simulink model "Ejercicio_Inestable_simu"  (R2021a)
settings: Solver=VariableStepAuto  StartTime=0.0  StopTime=10.0  RelTol=1e-3
values from neighbouring files (symbols this model uses):
  A = [-2 -1; 0 -4]    [Control_Integral.m]    (also in Controlabilidad.m = P.a; Ejemplo_filminas.m = SS.A; Ejercicio_Inestable.m = [100, 0; 160, 200]; Ejercicio_Valvulas.m = double(A))
  B = [1; 0]    [Control_Integral.m]    (also in Controlabilidad.m = P.b; Ejemplo_filminas.m = SS.B; Ejercicio_Inestable.m = [70; 160]; Ejercicio_Valvulas.m = double(B))
  C = [1 1]    [Control_Integral.m]    (also in Controlabilidad.m = P.c; Ejemplo_filminas.m = SS.C; Ejercicio_Inestable.m = [1, 1]; Ejercicio_Valvulas.m = double(C))
  D = 0    [Control_Integral.m]    (also in Controlabilidad.m = P.d; Ejemplo_filminas.m = SS.D; Ejercicio_Inestable.m = 1; Ejercicio_Valvulas.m = double(D))
  K = [p1-a1 p2-a2] * Wrm * inv(Wr)    [Controlabilidad.m]    (also in Ejemplo_filminas.m; Ejercicio_Inestable.m = [p1 - a1, p2 - a2] * Wrm * inv(Wr); Ejercicio_Valvulas.m = Ka(1:order(P)); realimentacion_ee.m = acker(A, B, [-10 -10]))
  K_nuevo = Ka(1:order(P))    [Ejemplo_filminas.m]    (also in Ejercicio_Inestable.m = Ka(1:2))
  kf = -1/(C*inv(A - B*K) * B)    [Controlabilidad.m]    (also in Ejemplo_filminas.m = -1/(Ccl * inv(Acl)*Bcl); Ejercicio_Inestable.m = 1/(-(C - D*K) * inv(A - B*K) * B + D); realimentacion_ee.m = 10)
  ki = 10    [Control_Integral.m]    (also in Ejemplo_filminas.m = - Ka(end); Ejercicio_Inestable.m = - Ka(end); Ejercicio_Valvulas.m = - Ka(end))
  L = zpk(ceros, polos, ganancia)    [Ejemplo_filminas.m]    (also in Ejercicio_Inestable.m = inv(Wo) * Wom * [l1 - a1; l2 - a2]; Observabilidad.m = [18; 99]; realimentacion_ee.m = [18; 99])
libraries: cstblocks x1
settings Model: Creator=Santiago  LastModifiedBy=Santiago

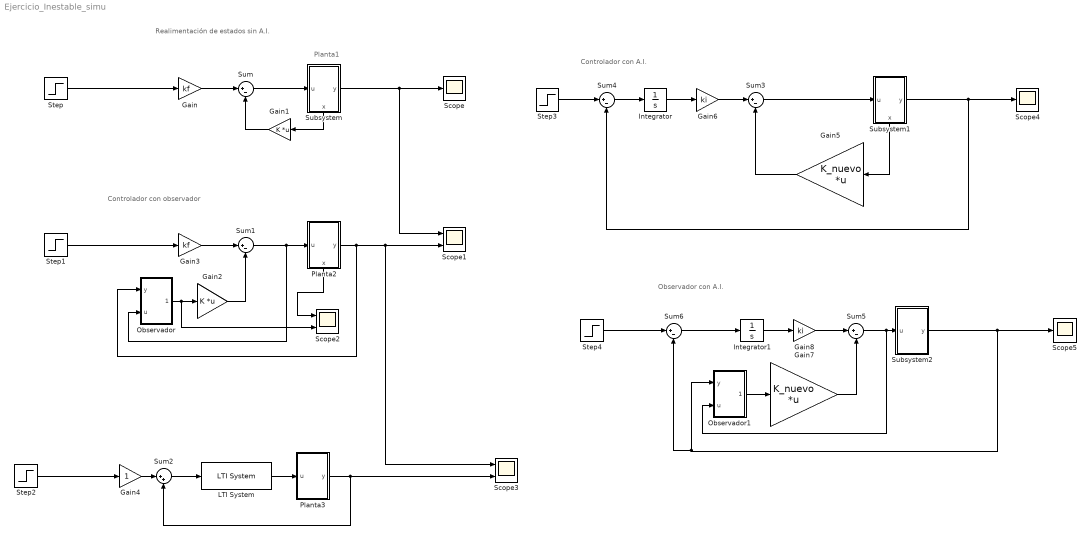
== system Ejercicio_Inestable_simu ==
  note: Observador con A.I.
  note: Controlador con A.I.
  note: Controlador con observador
  note: Realimentación de estados sin A.I.
  note: Planta1
  Gain : Gain  Gain=kf
  Gain1 : Gain  Gain=K  Multiplication=Matrix(K*u) (u vector)
  Gain2 : Gain  Gain=K  Multiplication=Matrix(K*u) (u vector)
  Gain3 : Gain  Gain=kf
  Gain4 : Gain
  Gain5 : Gain  Gain=K_nuevo  Multiplication=Matrix(K*u) (u vector)
  Gain6 : Gain  Gain=ki
  Gain7 : Gain  Gain=K_nuevo  Multiplication=Matrix(K*u) (u vector)
  Gain8 : Gain  Gain=ki
  Integrator : Integrator
  Integrator1 : Integrator
  LTI System : cstblocks/LTI System  sys=rsys  IC=[]
  Observador : Subsystem
  Observador1 : Subsystem
  Planta2 : Subsystem
      settings: PortSchema="{\"entries\":[{\"content\":{\"sides\":[{\"content\":{\"connectorIds\":[\"In1\"]},\"type\":\"ConnectorPlacement.EquallySpacedRectSide\",\"uuid\":\"42671557-4276-46e4-ad8c-bf843df94049\"},{\"content\":{\"connectorIds\":[\"Out1\"],\"side\":\"RIGHT\"},\"type\":\"ConnectorPlacement.EquallySpacedRectSide\",\"uuid\":\"cb79af1c-2dea-4382-b5e6-be31f4841be6\"},{\"content\":{\"connectorIds\":[],\"side\":\"TOP\"},\"type\":\"ConnectorPlacement.EquallySpacedRectSide\",\"uuid\":\"60d3f2a7-7810-4feb-a004-3efb06eed614\"},{\"content\":{\"connectorIds\":[\"Out2\"],\"side\":\"BOTTOM\"},\"type\":\"ConnectorPlacement.EquallySpacedRectSide\",\"uuid\":\"95700307-25c5-43ae-b0f1-57f7147fd329\"}]},\"type\":\"ConnectorPlacement.EquallySpacedConnector\",\"uuid\":\"693bd3af-f156-43df-9cc2-6d7d4d502922\"}],\"packageUris\":[\"http://schema.mathworks.com/mf0/Connector/R2020b\"],\"version\":\"1.0\"}"
  Planta3 : Subsystem
  Scope : Scope
  Scope1 : Scope  NumInputPorts=2
  Scope2 : Scope  NumInputPorts=2
  Scope3 : Scope  NumInputPorts=2
  Scope4 : Scope
  Scope5 : Scope
  Step{,1..4} (5 alike) : Step  SampleTime=0
  Subsystem : Subsystem
      settings: PortSchema="{\"entries\":[{\"content\":{\"sides\":[{\"content\":{\"connectorIds\":[\"In1\"]},\"type\":\"ConnectorPlacement.EquallySpacedRectSide\",\"uuid\":\"42671557-4276-46e4-ad8c-bf843df94049\"},{\"content\":{\"connectorIds\":[\"Out1\"],\"side\":\"RIGHT\"},\"type\":\"ConnectorPlacement.EquallySpacedRectSide\",\"uuid\":\"cb79af1c-2dea-4382-b5e6-be31f4841be6\"},{\"content\":{\"connectorIds\":[],\"side\":\"TOP\"},\"type\":\"ConnectorPlacement.EquallySpacedRectSide\",\"uuid\":\"60d3f2a7-7810-4feb-a004-3efb06eed614\"},{\"content\":{\"connectorIds\":[\"Out2\"],\"side\":\"BOTTOM\"},\"type\":\"ConnectorPlacement.EquallySpacedRectSide\",\"uuid\":\"9a7d0ef6-39ec-42a5-a60a-a43f88d1fbb1\"}]},\"type\":\"ConnectorPlacement.EquallySpacedConnector\",\"uuid\":\"693bd3af-f156-43df-9cc2-6d7d4d502922\"}],\"packageUris\":[\"http://schema.mathworks.com/mf0/Connector/R2020b\"],\"version\":\"1.0\"}"
  Subsystem1 : Subsystem
      settings: PortSchema="{\"entries\":[{\"content\":{\"sides\":[{\"content\":{\"connectorIds\":[\"In1\"]},\"type\":\"ConnectorPlacement.EquallySpacedRectSide\",\"uuid\":\"42671557-4276-46e4-ad8c-bf843df94049\"},{\"content\":{\"connectorIds\":[\"Out1\"],\"side\":\"RIGHT\"},\"type\":\"ConnectorPlacement.EquallySpacedRectSide\",\"uuid\":\"cb79af1c-2dea-4382-b5e6-be31f4841be6\"},{\"content\":{\"connectorIds\":[],\"side\":\"TOP\"},\"type\":\"ConnectorPlacement.EquallySpacedRectSide\",\"uuid\":\"60d3f2a7-7810-4feb-a004-3efb06eed614\"},{\"content\":{\"connectorIds\":[\"Out2\"],\"side\":\"BOTTOM\"},\"type\":\"ConnectorPlacement.EquallySpacedRectSide\",\"uuid\":\"9a7d0ef6-39ec-42a5-a60a-a43f88d1fbb1\"}]},\"type\":\"ConnectorPlacement.EquallySpacedConnector\",\"uuid\":\"693bd3af-f156-43df-9cc2-6d7d4d502922\"}],\"packageUris\":[\"http://schema.mathworks.com/mf0/Connector/R2020b\"],\"version\":\"1.0\"}"
  Subsystem2 : Subsystem
  Sum{,1,3..6} (6 alike) : Sum  Inputs=|+-
  Sum2 : Sum  Inputs=|++
  wires:
  Subsystem/1(y) -> Scope1/1, Scope/1
  Subsystem/2(x) -> Gain1/1
  Sum/1 -> Subsystem/1(u)
  Gain/1 -> Sum/1
  Step/1 -> Gain/1
  Gain1/1 -> Sum/2
  Observador/1(x_estim) -> Scope2/2, Gain2/1
  Gain2/1 -> Sum1/2
  Sum1/1 -> Observador/2(u), Planta2/1(u)
  Planta2/1(y) -> Observador/1(y), Scope3/1, Scope1/2
  Step1/1 -> Gain3/1
  Gain3/1 -> Sum1/1
  Planta2/2(x) -> Scope2/1
  Step2/1 -> Gain4/1
  Planta3/1(y) -> Sum2/2, Scope3/2
  Sum2/1 -> LTI System/1
  Gain4/1 -> Sum2/1
  LTI System/1 -> Planta3/1(u)
  Gain5/1 -> Sum3/2
  Gain6/1 -> Sum3/1
  Integrator/1 -> Gain6/1
  Sum4/1 -> Integrator/1
  Step3/1 -> Sum4/1
  Subsystem1/2(x) -> Gain5/1
  Sum3/1 -> Subsystem1/1(u)
  Subsystem1/1(y) -> Sum4/2, Scope4/1
  Gain8/1 -> Sum5/1
  Integrator1/1 -> Gain8/1
  Observador1/1(x_estim) -> Gain7/1
  Gain7/1 -> Sum5/2
  Sum5/1 -> Observador1/2(u), Subsystem2/1(u)
  Subsystem2/1(y) -> Sum6/2, Observador1/1(y), Scope5/1
  Step4/1 -> Sum6/1
  Sum6/1 -> Integrator1/1

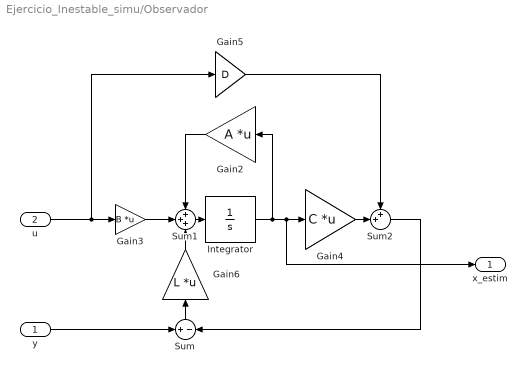
== system Ejercicio_Inestable_simu/Observador ==
  y : Inport
  u : Inport  Port=2
  Gain2 : Gain  Gain=A  Multiplication=Matrix(K*u) (u vector)
  Gain3 : Gain  Gain=B  Multiplication=Matrix(K*u)
  Gain4 : Gain  Gain=C  Multiplication=Matrix(K*u) (u vector)
  Gain5 : Gain  Gain=D
  Gain6 : Gain  Gain=L  Multiplication=Matrix(K*u) (u vector)
  Integrator : Integrator
  Sum : Sum  Inputs=+|-
  Sum1 : Sum  Inputs=+++
  Sum2 : Sum  Inputs=++|
  x_estim : Outport
  wires:
  Sum2/1 -> Sum/2
  Integrator/1 -> Gain4/1, x_estim/1, Gain2/1
  Gain5/1 -> Sum2/1
  Gain3/1 -> Sum1/2
  Gain4/1 -> Sum2/2
  u/1 -> Gain5/1, Gain3/1
  Sum1/1 -> Integrator/1
  Gain2/1 -> Sum1/1
  y/1 -> Sum/1
  Sum/1 -> Gain6/1
  Gain6/1 -> Sum1/3

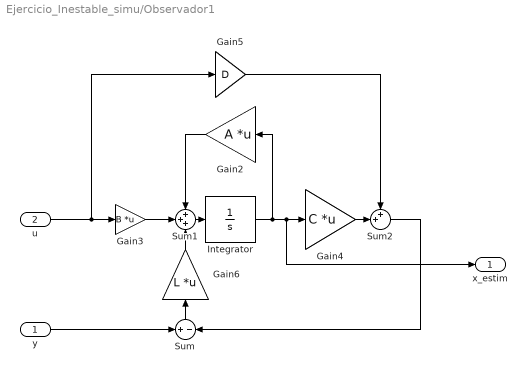
== system Ejercicio_Inestable_simu/Observador1 ==
  y : Inport
  u : Inport  Port=2
  Gain2 : Gain  Gain=A  Multiplication=Matrix(K*u) (u vector)
  Gain3 : Gain  Gain=B  Multiplication=Matrix(K*u)
  Gain4 : Gain  Gain=C  Multiplication=Matrix(K*u) (u vector)
  Gain5 : Gain  Gain=D
  Gain6 : Gain  Gain=L  Multiplication=Matrix(K*u) (u vector)
  Integrator : Integrator
  Sum : Sum  Inputs=+|-
  Sum1 : Sum  Inputs=+++
  Sum2 : Sum  Inputs=++|
  x_estim : Outport
  wires:
  Sum2/1 -> Sum/2
  Integrator/1 -> Gain4/1, x_estim/1, Gain2/1
  Gain5/1 -> Sum2/1
  Gain3/1 -> Sum1/2
  Gain4/1 -> Sum2/2
  u/1 -> Gain5/1, Gain3/1
  Sum1/1 -> Integrator/1
  Gain2/1 -> Sum1/1
  y/1 -> Sum/1
  Sum/1 -> Gain6/1
  Gain6/1 -> Sum1/3

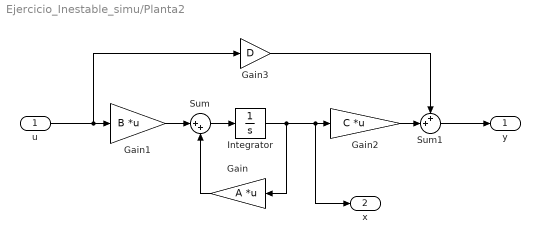
== system Ejercicio_Inestable_simu/Planta2 ==
  u : Inport
  Gain : Gain  Gain=A  Multiplication=Matrix(K*u) (u vector)
  Gain1 : Gain  Gain=B  Multiplication=Matrix(K*u) (u vector)
  Gain2 : Gain  Gain=C  Multiplication=Matrix(K*u) (u vector)
  Gain3 : Gain  Gain=D
  Integrator : Integrator
  Sum : Sum  Inputs=|++
  Sum1 : Sum  Inputs=++|
  y : Outport
  x : Outport  Port=2
  wires:
  Integrator/1 -> x/1, Gain2/1, Gain/1
  Gain/1 -> Sum/2
  Sum/1 -> Integrator/1
  Gain2/1 -> Sum1/2
  u/1 -> Gain3/1, Gain1/1
  Sum1/1 -> y/1
  Gain3/1 -> Sum1/1
  Gain1/1 -> Sum/1

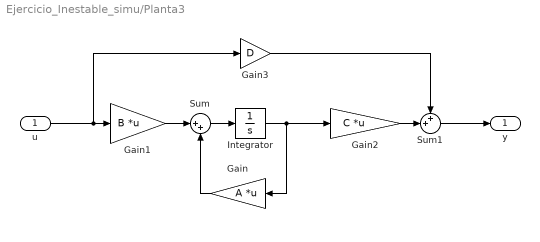
== system Ejercicio_Inestable_simu/Planta3 ==
  u : Inport
  Gain : Gain  Gain=A  Multiplication=Matrix(K*u) (u vector)
  Gain1 : Gain  Gain=B  Multiplication=Matrix(K*u) (u vector)
  Gain2 : Gain  Gain=C  Multiplication=Matrix(K*u) (u vector)
  Gain3 : Gain  Gain=D
  Integrator : Integrator
  Sum : Sum  Inputs=|++
  Sum1 : Sum  Inputs=++|
  y : Outport
  wires:
  Integrator/1 -> Gain2/1, Gain/1
  Gain/1 -> Sum/2
  Sum/1 -> Integrator/1
  Gain2/1 -> Sum1/2
  u/1 -> Gain3/1, Gain1/1
  Sum1/1 -> y/1
  Gain3/1 -> Sum1/1
  Gain1/1 -> Sum/1

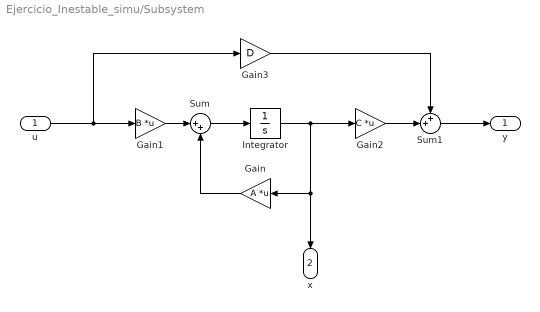
== system Ejercicio_Inestable_simu/Subsystem ==
  u : Inport
  Gain : Gain  Gain=A  Multiplication=Matrix(K*u) (u vector)
  Gain1 : Gain  Gain=B  Multiplication=Matrix(K*u) (u vector)
  Gain2 : Gain  Gain=C  Multiplication=Matrix(K*u) (u vector)
  Gain3 : Gain  Gain=D
  Integrator : Integrator
  Sum : Sum  Inputs=|++
  Sum1 : Sum  Inputs=++|
  y : Outport
  x : Outport  Port=2
  wires:
  Integrator/1 -> Gain/1, x/1, Gain2/1
  Gain/1 -> Sum/2
  Sum/1 -> Integrator/1
  Gain2/1 -> Sum1/2
  u/1 -> Gain3/1, Gain1/1
  Sum1/1 -> y/1
  Gain3/1 -> Sum1/1
  Gain1/1 -> Sum/1

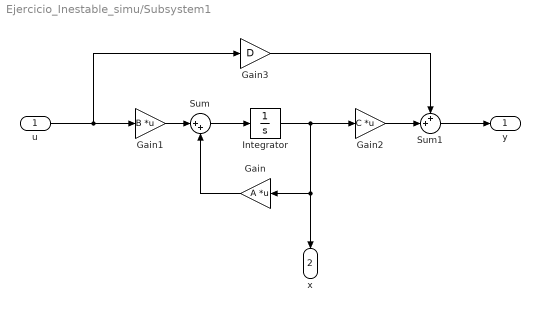
== system Ejercicio_Inestable_simu/Subsystem1 ==
  u : Inport
  Gain : Gain  Gain=A  Multiplication=Matrix(K*u) (u vector)
  Gain1 : Gain  Gain=B  Multiplication=Matrix(K*u) (u vector)
  Gain2 : Gain  Gain=C  Multiplication=Matrix(K*u) (u vector)
  Gain3 : Gain  Gain=D
  Integrator : Integrator
  Sum : Sum  Inputs=|++
  Sum1 : Sum  Inputs=++|
  y : Outport
  x : Outport  Port=2
  wires:
  Integrator/1 -> Gain/1, x/1, Gain2/1
  Gain/1 -> Sum/2
  Sum/1 -> Integrator/1
  Gain2/1 -> Sum1/2
  u/1 -> Gain3/1, Gain1/1
  Sum1/1 -> y/1
  Gain3/1 -> Sum1/1
  Gain1/1 -> Sum/1

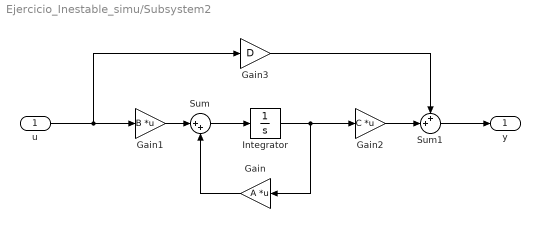
== system Ejercicio_Inestable_simu/Subsystem2 ==
  u : Inport
  Gain : Gain  Gain=A  Multiplication=Matrix(K*u) (u vector)
  Gain1 : Gain  Gain=B  Multiplication=Matrix(K*u) (u vector)
  Gain2 : Gain  Gain=C  Multiplication=Matrix(K*u) (u vector)
  Gain3 : Gain  Gain=D
  Integrator : Integrator
  Sum : Sum  Inputs=|++
  Sum1 : Sum  Inputs=++|
  y : Outport
  wires:
  Integrator/1 -> Gain/1, Gain2/1
  Gain/1 -> Sum/2
  Sum/1 -> Integrator/1
  Gain2/1 -> Sum1/2
  u/1 -> Gain3/1, Gain1/1
  Sum1/1 -> y/1
  Gain3/1 -> Sum1/1
  Gain1/1 -> Sum/1
